simulink subsystem "BatterySoCEstimation"  (R2024b)
settings: Solver=VariableStepAuto  StartTime=0.0  StopTime=10.0  RelTol=1e-3
undefined symbols (not defined in the file): Batt_Em0_LUT, Batt_MaxCoulomb, Batt_nrCellSeries, Batt_SoC_LUT, DiscIntNeverNeededParam, SEPIC_Efficiency
settings Model: DefaultTestHarness=Supervisory_Logic_Harness  Creator=vlenzi  LastModifiedBy=vlenzi
settings RTWCC: GPUComputeCapability=3.5

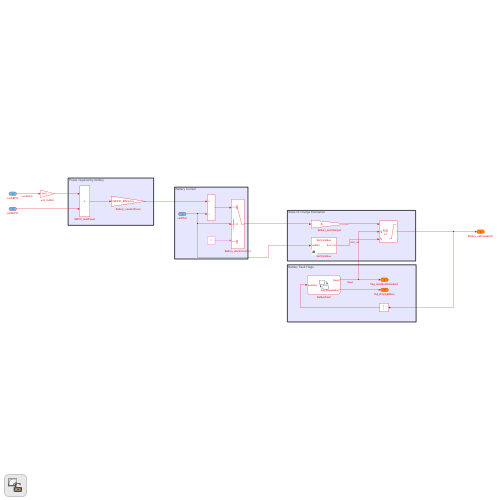
[thumbnail: Simulink's stored preview of the top-level diagram]
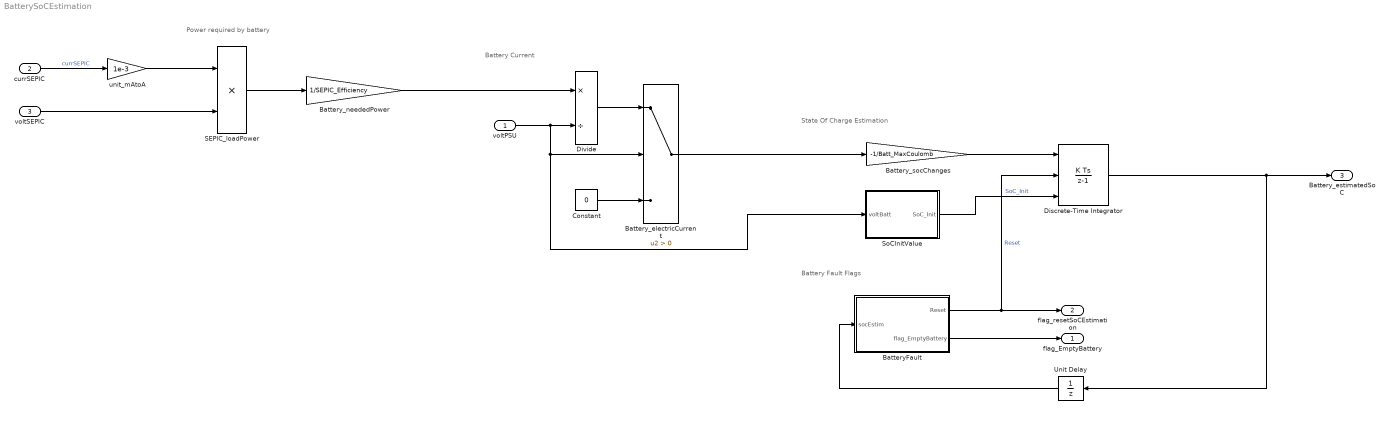
== system BatterySoCEstimation ==
  note: State Of Charge Estimation
  note: Power required by battery
  note: Battery Fault Flags
  note: Battery Current
  voltPSU : Inport  OutDataTypeStr=single  Unit=V  PortDimensions=1
  currSEPIC : Inport  Port=2  OutDataTypeStr=single  Unit=mA  PortDimensions=1
  voltSEPIC : Inport  Port=3
  BatteryFault : Stateflow chart  TreatAsAtomicUnit=on
  Battery_electricCurrent : Switch  Criteria=u2 > Threshold  SaturateOnIntegerOverflow=off  InputSameDT=off
  Battery_neededPower : Gain  Gain=1/SEPIC_Efficiency
  Battery_socChanges : Gain  Gain=-1/Batt_MaxCoulomb
  Constant : Constant  Value=0  OutDataTypeStr=single  SampleTime=-1
  Discrete-Time Integrator : DiscreteIntegrator  ExternalReset=falling  InitialConditionSource=external  SampleTime=-1  OutDataTypeStr=single  LimitOutput=on  UpperSaturationLimit=1  LowerSaturationLimit=0  ICPrevOutput=DiscIntNeverNeededParam  ICPrevScaledInput=DiscIntNeverNeededParam
  Divide : Product  Inputs=*/
  SEPIC_loadPower : Product
  SoCInitValue : Subsystem  Variant=on  VariantControlMode=label  VariantControl=Variant1  LabelModeActiveChoice=Simulink_LUT
  Unit Delay : UnitDelay  SampleTime=-1  HasFrameUpgradeWarning=on
  unit_mAtoA : Gain  Gain=1e-3
  flag_EmptyBattery : Outport  OutDataTypeStr=boolean  Unit=1  PortDimensions=1  VectorParamsAs1DForOutWhenUnconnected=off
  flag_resetSoCEstimation : Outport  Port=2  OutDataTypeStr=boolean  Unit=1  PortDimensions=1  VectorParamsAs1DForOutWhenUnconnected=off
  Battery_estimatedSoC : Outport  Port=3  OutDataTypeStr=single  Unit=1  PortDimensions=1  VectorParamsAs1DForOutWhenUnconnected=off
  wires:
  Constant/1 -> Battery_electricCurrent/3
  Discrete-Time Integrator/1 -> Battery_estimatedSoC/1, Unit Delay/1
  unit_mAtoA/1 -> SEPIC_loadPower/1
  Battery_electricCurrent/1 -> Battery_socChanges/1
  Divide/1 -> Battery_electricCurrent/1
  voltPSU/1 -> SoCInitValue/1("voltBatt "), Battery_electricCurrent/2, Divide/2
  BatteryFault/1(Reset) -> flag_resetSoCEstimation/1, Discrete-Time Integrator/2  "Reset"
  Battery_neededPower/1 -> Divide/1
  Unit Delay/1 -> BatteryFault/1(socEstim)
  BatteryFault/2(flag_EmptyBattery) -> flag_EmptyBattery/1
  SEPIC_loadPower/1 -> Battery_neededPower/1
  voltSEPIC/1 -> SEPIC_loadPower/2
  currSEPIC/1 -> unit_mAtoA/1  "currSEPIC"
  SoCInitValue/1(" SoC_Init") -> Discrete-Time Integrator/3  "SoC_Init"
  Battery_socChanges/1 -> Discrete-Time Integrator/1

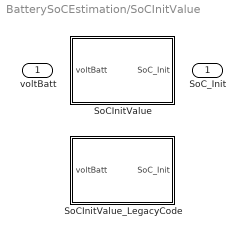
== system BatterySoCEstimation/SoCInitValue ==
  "voltBatt " : Inport
  SoCInitValue : Subsystem  VariantControl=Simulink_LUT
  SoCInitValue_LegacyCode : Subsystem  VariantControl=CCode_LUT
  " SoC_Init" : Outport  VectorParamsAs1DForOutWhenUnconnected=off

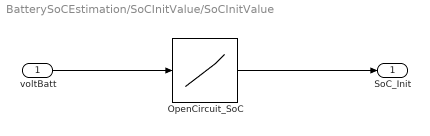
== system BatterySoCEstimation/SoCInitValue/SoCInitValue ==
  voltBatt : Inport
  OpenCircuit_SoC : Lookup_n-D  NumberOfTableDimensions=1  BreakpointsForDimension1=Batt_Em0_LUT*Batt_nrCellSeries  Table=Batt_SoC_LUT  InternalRulePriority=Speed  OutMin=0  OutMax=1  RndMeth=Simplest
  SoC_Init : Outport  VectorParamsAs1DForOutWhenUnconnected=off
  wires:
  OpenCircuit_SoC/1 -> SoC_Init/1
  voltBatt/1 -> OpenCircuit_SoC/1

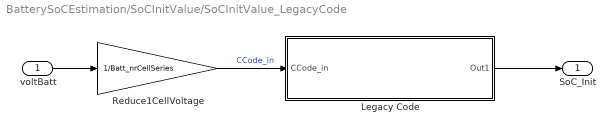
== system BatterySoCEstimation/SoCInitValue/SoCInitValue_LegacyCode ==
  voltBatt : Inport
  Legacy Code : Subsystem
  Reduce1CellVoltage : Gain  Gain=1/Batt_nrCellSeries
  SoC_Init : Outport  VectorParamsAs1DForOutWhenUnconnected=off
  wires:
  voltBatt/1 -> Reduce1CellVoltage/1
  Reduce1CellVoltage/1 -> Legacy Code/1(CCode_in)  "CCode_in"
  Legacy Code/1(Out1) -> SoC_Init/1

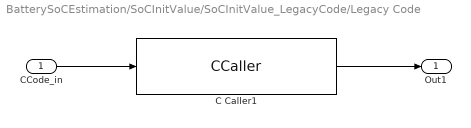
== system BatterySoCEstimation/SoCInitValue/SoCInitValue_LegacyCode/Legacy Code ==
  CCode_in : Inport
  C Caller1 : CCaller  FunctionName=EmLiIon_LUT
  Out1 : Outport  VectorParamsAs1DForOutWhenUnconnected=off
  wires:
  C Caller1/1 -> Out1/1
  CCode_in/1 -> C Caller1/1

== stateflow chart BatterySoCEstimation/BatteryFault ==
  state Resetting_Integrator
    en:Reset=true;
    flag_EmptyBattery=false;
    ex:Reset=false;
  state running
    state Normal
      du:flag_EmptyBattery=false;
    state Battery_Empty
      en:flag_EmptyBattery=true;
    (default) -> Normal
    Normal -> Battery_Empty : [socEstim<=0.05]
  (default) -> Resetting_Integrator
  Resetting_Integrator -> running : [after(0.5,sec)]
  data: Reset output boolean; socEstim input single size=1; flag_EmptyBattery output
